simulink model "System_A"  (R2018a)
settings: Solver=VariableStepAuto  StartTime=0.0  StopTime=5  RelTol=1e-3
libraries: dspsrcs4 x1
settings Model: Creator=Risky Jr  LastModifiedBy=Risky Jr

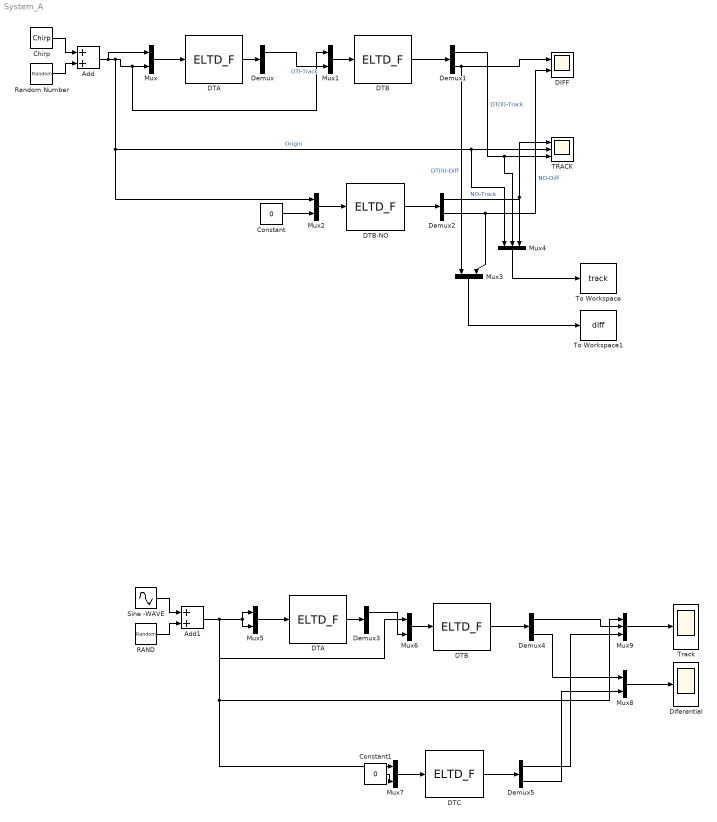
== system System_A ==
  Add : Sum
  Add1 : Sum
  Chirp : dspsrcs4/Chirp  sweep=Swept cosine  mode=Unidirectional  f0=1  f1=5  t1=5  Tsweep=5  phase=1.5*pi  Ts=0.001  spf=1  datatype=Double  OutputFrames=off
      settings: SourceProductName=DSP System Toolbox
  Constant : Constant  Value=0
  Constant1 : Constant  Value=0
  DIFF : Scope  NumInputPorts=2
  DTA : S-Function  FunctionName=ELTD_F  Parameters=2.2,1.3,15,5  SFunctionDeploymentMode=off  EnableBusSupport=off
  "DTA " : S-Function  FunctionName=ELTD_F  Parameters=2.2,1.3,15,5  SFunctionDeploymentMode=off  EnableBusSupport=off
  DTB : S-Function  FunctionName=ELTD_F  Parameters=2.2,2.8,30,40  SFunctionDeploymentMode=off  EnableBusSupport=off
  "DTB " : S-Function  FunctionName=ELTD_F  Parameters=2.2,2.8,30,40  SFunctionDeploymentMode=off  EnableBusSupport=off
  DTB-NO : S-Function  FunctionName=ELTD_F  Parameters=2.2,2.8,30,40  SFunctionDeploymentMode=off  EnableBusSupport=off
  DTC : S-Function  FunctionName=ELTD_F  Parameters=2.2,2.8,30,40  SFunctionDeploymentMode=off  EnableBusSupport=off
  Demux{,1..5} (6 alike) : Demux  Outputs=2
  Diferential : Scope
  Mux{,1..3,5..8} (8 alike) : Mux  Inputs=2
  Mux4 : Mux  Inputs=3
  Mux9 : Mux  Inputs=3
  RAND : RandomNumber  Variance=0.01  SampleTime=0.001
  Random Number : RandomNumber  Variance=0.01  SampleTime=0.001
  Sine -WAVE : Sin  SampleTime=0
  TRACK : Scope  NumInputPorts=3
  To Workspace : ToWorkspace  VariableName=track  SampleTime=-1
      settings: Save2DSignal=2-D array (concatenate along first dimension)
  To Workspace1 : ToWorkspace  VariableName=diff  SampleTime=-1
      settings: Save2DSignal=2-D array (concatenate along first dimension)
  Track : Scope
  wires:
  "DTA "/1 -> Demux/1
  "DTB "/1 -> Demux1/1
  Chirp/1 -> Add/1
  Random Number/1 -> Add/2
  Add/1 -> Mux/1, Mux2/1, Mux4/1, TRACK/2, Mux1/1, Mux/2  "Origin"
  Mux/1 -> "DTA "/1
  Mux1/1 -> "DTB "/1
  Demux1/1 -> Mux4/2, TRACK/3  "DT(II)-Track"
  Mux2/1 -> DTB-NO/1
  DTB-NO/1 -> Demux2/1
  Demux1/2 -> Mux3/1, DIFF/1  "DT(II)-Diff"
  Demux2/1 -> Mux4/3, TRACK/1  "NO-Track"
  Demux2/2 -> Mux3/2, DIFF/2  "NO-Diff"
  Constant/1 -> Mux2/2
  Demux/1 -> Mux1/2  "DTI-Track"
  Mux4/1 -> To Workspace/1
  Mux3/1 -> To Workspace1/1
  DTC/1 -> Demux5/1
  Demux3/1 -> Mux6/2
  Demux5/2 -> Mux8/2
  Mux9/1 -> Track/1
  Demux5/1 -> Mux9/3
  Constant1/1 -> Mux7/2
  Demux4/1 -> Mux9/2
  Sine -WAVE/1 -> Add1/1
  Demux4/2 -> Mux8/1
  Mux8/1 -> Diferential/1
  RAND/1 -> Add1/2
  Mux5/1 -> DTA/1
  DTB/1 -> Demux4/1
  Mux7/1 -> DTC/1
  DTA/1 -> Demux3/1
  Mux6/1 -> DTB/1
  Add1/1 -> Mux5/2, Mux5/1, Mux7/1, Mux9/1, Mux6/1
